simulink model "MODELOENTERO"  (R2017b)
settings: Solver=ode4  StartTime=0  StopTime=500  FixedStep=0.1  RelTol=1e-3
settings Model: Creator=Daples  LastModifiedBy=Daples

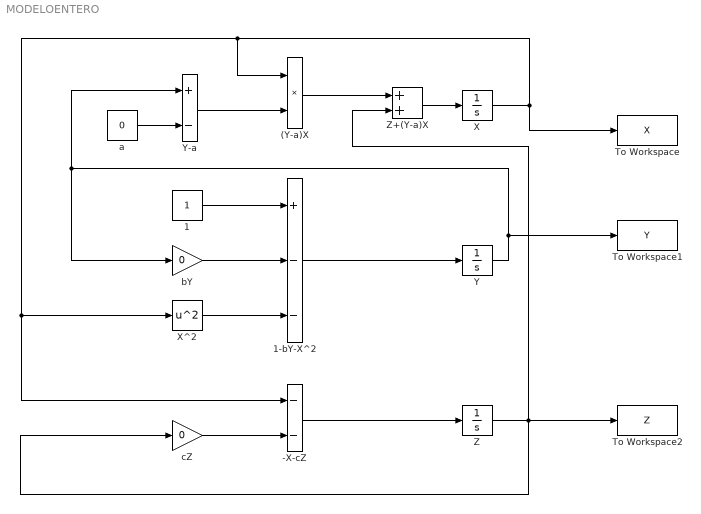
== system MODELOENTERO ==
  (Y-a)X : Product
  -X-cZ : Sum  Inputs=--
  "1 " : Constant
  1-bY-X^2 : Sum  Inputs=+--
  To Workspace : ToWorkspace  VariableName=X  SampleTime=-1
      settings: Save2DSignal=2-D array (concatenate along first dimension)
  To Workspace1 : ToWorkspace  VariableName=Y  SampleTime=-1
      settings: Save2DSignal=2-D array (concatenate along first dimension)
  To Workspace2 : ToWorkspace  VariableName=Z  SampleTime=-1
      settings: Save2DSignal=2-D array (concatenate along first dimension)
  X : Integrator
  X^2 : Math  Operator=square  SaturateOnIntegerOverflow=on
  Y : Integrator
  Y-a : Sum  Inputs=+-
  Z : Integrator  InitialCondition=1.6
  Z+(Y-a)X : Sum
  a : Constant  Value=0
  bY : Gain  Gain=0
  cZ : Gain  Gain=0
  wires:
  Z+(Y-a)X/1 -> X/1
  (Y-a)X/1 -> Z+(Y-a)X/1
  X/1 -> -X-cZ/1, X^2/1, (Y-a)X/1, To Workspace/1
  Y/1 -> bY/1, Y-a/1, To Workspace1/1
  a/1 -> Y-a/2
  Y-a/1 -> (Y-a)X/2
  1-bY-X^2/1 -> Y/1
  "1 "/1 -> 1-bY-X^2/1
  bY/1 -> 1-bY-X^2/2
  X^2/1 -> 1-bY-X^2/3
  -X-cZ/1 -> Z/1
  cZ/1 -> -X-cZ/2
  Z/1 -> To Workspace2/1, cZ/1, Z+(Y-a)X/2
